simulink model "xiti4_131"  (Simulink 8.3)
settings: Solver=ode45  SolverMode=SingleTasking  StartTime=0.0  StopTime=100  FixedStep=0.25  RelTol=1e-3
values from neighbouring files (symbols this model uses):
  kd = kp*pi/(4*wr)    [xiti4_13Dm.m]    (also in xiti4_13Dm1.m)
  ki = kp*wr/pi    [xiti4_13Dm.m]    (also in xiti4_13Dm1.m)
  kp = 0.6*kr    [xiti4_13Dm.m]    (also in xiti4_13Dm1.m)
undefined symbols (not defined in the file or in its folder): DiscIntNeverNeededParam
settings Model: Creator=sony  LastModifiedBy=sony  ExtModeTrigMode=oneshot  ExtModeArmWhenConnect=off
settings DataIOCC: LimitDataPoints=off  SignalLoggingName=sigsOut
settings OptimizationCC: BooleanDataType=off
settings DebuggingCC: SaveWithParameterizedLinksMsg=none  SignalResolutionControl=TryResolveAllWithWarning  SolverPrmCheckMsg=none  MultiTaskDSMMsg=warning  MultiTaskCondExecSysMsg=none  StateNameClashWarn=none  StrictBusMsg=None
settings HardwareCC: TargetUnknown=on
settings RTWCC: IncludeERTFirstTime=on

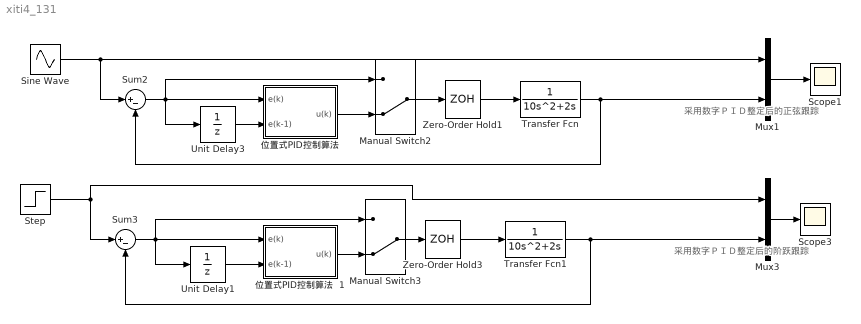
== system xiti4_131 ==
  note: 采用数字ＰＩＤ整定后的正弦跟踪
  note: 采用数字ＰＩＤ整定后的阶跃跟踪
  Manual Switch2 : ManualSwitch  CurrentSetting=0
  Manual Switch3 : ManualSwitch  CurrentSetting=0
  Mux1 : Mux  Inputs=2
  Mux3 : Mux  Inputs=2
  Scope1 : Scope
      settings: YMin=-3.5  YMax=1  MaxDataPoints=500000
  Scope3 : Scope
      settings: YMin=-3.5  YMax=1  SaveName=ScopeData2  MaxDataPoints=500000
  Sine Wave : Sin  Amplitude=0.5  Frequency=0.05*pi  SampleTime=0
  Step : Step  Time=0  SampleTime=0
  Sum2 : Sum  Inputs=|+-  SaturateOnIntegerOverflow=on
  Sum3 : Sum  Inputs=|+-  SaturateOnIntegerOverflow=on
  Transfer Fcn : TransferFcn  Denominator=[10 2 0]
  Transfer Fcn1 : TransferFcn  Denominator=[10 2 0]
  Unit Delay1 : UnitDelay  SampleTime=0.25
  Unit Delay3 : UnitDelay  SampleTime=0.25
  Zero-Order Hold1 : ZeroOrderHold  SampleTime=0.25
  Zero-Order Hold3 : ZeroOrderHold  SampleTime=0.25
  "位置式PID控制算法  " : Subsystem
  位置式PID控制算法  1 : Subsystem
  wires:
  Sine Wave/1 -> Sum2/1, Mux1/1
  Mux1/1 -> Scope1/1
  Transfer Fcn/1 -> Sum2/2, Mux1/2
  Unit Delay3/1 -> "位置式PID控制算法  "/2(e(k-1))
  Sum2/1 -> "位置式PID控制算法  "/1(e(k)), Manual Switch2/1, Unit Delay3/1
  "位置式PID控制算法  "/1(u(k)) -> Manual Switch2/2
  Zero-Order Hold1/1 -> Transfer Fcn/1
  Manual Switch2/1 -> Zero-Order Hold1/1
  Step/1 -> Sum3/1, Mux3/1
  Mux3/1 -> Scope3/1
  Transfer Fcn1/1 -> Sum3/2, Mux3/2
  Unit Delay1/1 -> 位置式PID控制算法  1/2(e(k-1))
  Sum3/1 -> Manual Switch3/1, Unit Delay1/1, 位置式PID控制算法  1/1(e(k))
  位置式PID控制算法  1/1(u(k)) -> Manual Switch3/2
  Zero-Order Hold3/1 -> Transfer Fcn1/1
  Manual Switch3/1 -> Zero-Order Hold3/1

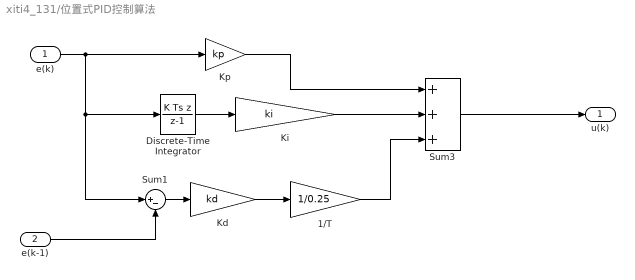
== system xiti4_131/位置式PID控制算法   ==
  e(k) : Inport
  e(k-1) : Inport  Port=2
  1/T : Gain  Gain=1/0.25  SaturateOnIntegerOverflow=on  OutDataTypeStr=Inherit: Same as input  ParamDataTypeStr=Inherit: Same as input
  Discrete-Time Integrator : DiscreteIntegrator  IntegratorMethod=Integration: Backward Euler  SampleTime=0.25  ICPrevOutput=DiscIntNeverNeededParam  ICPrevScaledInput=DiscIntNeverNeededParam
  Kd : Gain  Gain=kd  SaturateOnIntegerOverflow=on  OutDataTypeStr=Inherit: Same as input  ParamDataTypeStr=Inherit: Same as input
  Ki : Gain  Gain=ki  SaturateOnIntegerOverflow=on  OutDataTypeStr=Inherit: Same as input  ParamDataTypeStr=Inherit: Same as input
  Kp : Gain  Gain=kp  SaturateOnIntegerOverflow=on  OutDataTypeStr=Inherit: Same as input  ParamDataTypeStr=Inherit: Same as input
  Sum1 : Sum  Inputs=|+-  SaturateOnIntegerOverflow=on
  Sum3 : Sum  Inputs=+++  SaturateOnIntegerOverflow=on
  u(k) : Outport
  wires:
  e(k-1)/1 -> Sum1/2
  1/T/1 -> Sum3/3
  Kd/1 -> 1/T/1
  Sum3/1 -> u(k)/1
  Ki/1 -> Sum3/2
  Kp/1 -> Sum3/1
  e(k)/1 -> Sum1/1, Discrete-Time Integrator/1, Kp/1
  Sum1/1 -> Kd/1
  Discrete-Time Integrator/1 -> Ki/1

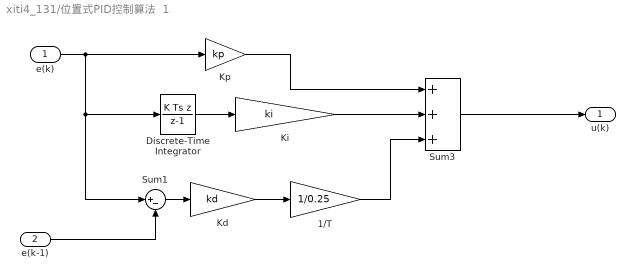
== system xiti4_131/位置式PID控制算法  1 ==
  e(k) : Inport
  e(k-1) : Inport  Port=2
  1/T : Gain  Gain=1/0.25  SaturateOnIntegerOverflow=on  OutDataTypeStr=Inherit: Same as input  ParamDataTypeStr=Inherit: Same as input
  Discrete-Time Integrator : DiscreteIntegrator  IntegratorMethod=Integration: Backward Euler  SampleTime=0.25  ICPrevOutput=DiscIntNeverNeededParam  ICPrevScaledInput=DiscIntNeverNeededParam
  Kd : Gain  Gain=kd  SaturateOnIntegerOverflow=on  OutDataTypeStr=Inherit: Same as input  ParamDataTypeStr=Inherit: Same as input
  Ki : Gain  Gain=ki  SaturateOnIntegerOverflow=on  OutDataTypeStr=Inherit: Same as input  ParamDataTypeStr=Inherit: Same as input
  Kp : Gain  Gain=kp  SaturateOnIntegerOverflow=on  OutDataTypeStr=Inherit: Same as input  ParamDataTypeStr=Inherit: Same as input
  Sum1 : Sum  Inputs=|+-  SaturateOnIntegerOverflow=on
  Sum3 : Sum  Inputs=+++  SaturateOnIntegerOverflow=on
  u(k) : Outport
  wires:
  e(k-1)/1 -> Sum1/2
  1/T/1 -> Sum3/3
  Kd/1 -> 1/T/1
  Sum3/1 -> u(k)/1
  Ki/1 -> Sum3/2
  Kp/1 -> Sum3/1
  e(k)/1 -> Sum1/1, Discrete-Time Integrator/1, Kp/1
  Sum1/1 -> Kd/1
  Discrete-Time Integrator/1 -> Ki/1
